simulink model "Hilaire07Martinez"  (R2023b)
settings: Solver=ode4  StartTime=t(1)  StopTime=t(end)+dt  FixedStep=dt  RelTol=1e-3
values from neighbouring files (symbols this model uses):
  nInitial = initial_conditions(3)    [hilaire07martinez_simulink.m]    (also in jewett99_simulink.m)
  processLParams = [a0, p, beta, G, I0]    [hilaire07martinez_simulink.m]    (also in jewett99_simulink.m)
  processPParams = [mu, k, q, kc, tau]    [hilaire07martinez_simulink.m]    (also in jewett99_simulink.m)
  xInitial = [initial_conditions ... (first row only)    [gois09_simulink.m]    (also in hilaire07martinez_simulink.m = initial_conditions(1:2); jewett99_simulink.m = initial_conditions(1:2); ryzhii14_simulink.m; sinoatrial_simulink.m = initial_conditions)
settings Model: Creator=chukw  LastModifiedBy=chukw

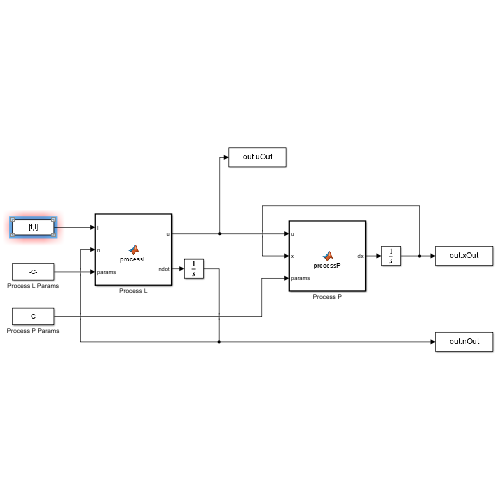
[thumbnail: Simulink's stored preview of the top-level diagram]
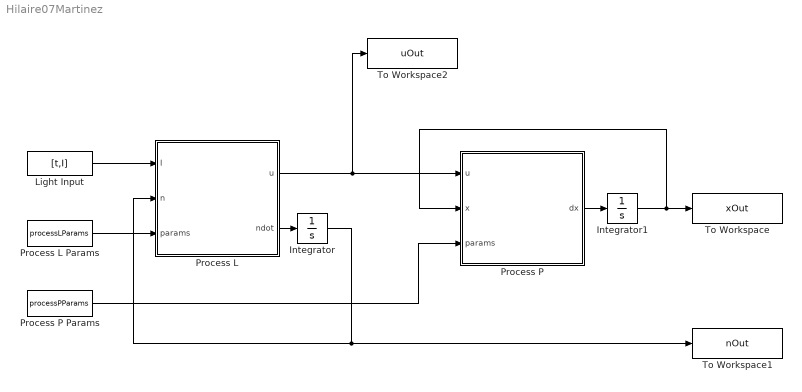
== system Hilaire07Martinez ==
  Integrator : Integrator  InitialCondition=nInitial
  Integrator1 : Integrator  InitialCondition=xInitial
  Light Input : FromWorkspace  VariableName=[t,I]
  Process L : MATLAB Function  TreatAsAtomicUnit=on
  Process L Params : Constant  Value=processLParams
  Process P : MATLAB Function  TreatAsAtomicUnit=on
  Process P Params : Constant  Value=processPParams
  To Workspace : ToWorkspace  VariableName=xOut  SampleTime=-1
  To Workspace1 : ToWorkspace  VariableName=nOut  SampleTime=-1
  To Workspace2 : ToWorkspace  VariableName=uOut  SampleTime=-1
  wires:
  Integrator1/1 -> To Workspace/1, Process P/2(x)
  Process L/1(u) -> To Workspace2/1, Process P/1(u)
  Integrator/1 -> To Workspace1/1, Process L/2(n)
  Process L Params/1 -> Process L/3(params)
  Process P/1(dx) -> Integrator1/1
  Light Input/1 -> Process L/1(I)
  Process P Params/1 -> Process P/3(params)
  Process L/2(ndot) -> Integrator/1

== matlab function Hilaire07Martinez/Process P ==
  data: u input; dx output; x input; params input
function dx = processP(u,x,params)

    mu = params(1);
    k = params(2);
    q = params(3);
    kc = params(4);
    tau = params(5);

    B = u*(1-0.4*x(1))*(1-kc*x(2));

    dx = zeros(2,1);
    dx(1) = (pi/12)*(x(2) + mu*((x(1)/3)+(4*x(1)^3/3)-(256*x(1)^7/105)) + B);
    dx(2) = (pi/12)*(q*x(2)*B - x(1)*((24/0.99729/tau)^2 + k*B));
end

== matlab function Hilaire07Martinez/Process L ==
  data: I input; u output; n input; ndot output; params input
function [u, ndot] = processL(I,n,params)

    a0 = params(1);
    p = params(2);
    beta = params(3);
    G = params(4);
    I0 = params(5);
    
    alpha = (a0*(I/I0)^p)*(I/(I+100));
    
    ndot = 60*((alpha*(1-n)) - (beta*n));
    
    u = G*alpha*(1-n);
end
